simulink model "Desired_path_Block"  (R2022a)
settings: Solver=VariableStepAuto  StartTime=0.0  StopTime=10.0  RelTol=1e-3
settings Model: Creator=radha  LastModifiedBy=radha

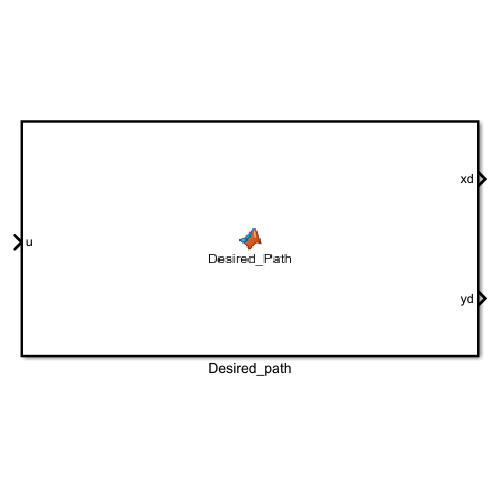
[thumbnail: Simulink's stored preview of the top-level diagram]
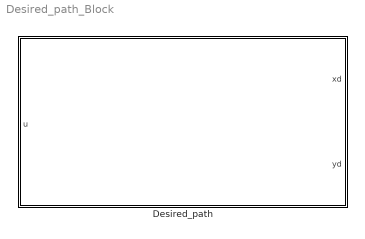
== system Desired_path_Block ==
  Desired_path : MATLAB Function  TreatAsAtomicUnit=on

== matlab function Desired_path_Block/Desired_path ==
  data: u input; xd output; yd output
function [xd, yd] = Desired_Path(u)

xd = 1+0.5*sin((2*pi/5)*u+pi/2);
yd = 1+0.5*cos((2*pi/5)*u+pi/2);
